simulink model "iface"  (R2018b)
settings: Solver=FixedStepDiscrete  StartTime=0.0  StopTime=10.0  RelTol=1e-3
settings Model: Creator=matlab  LastModifiedBy=matlab

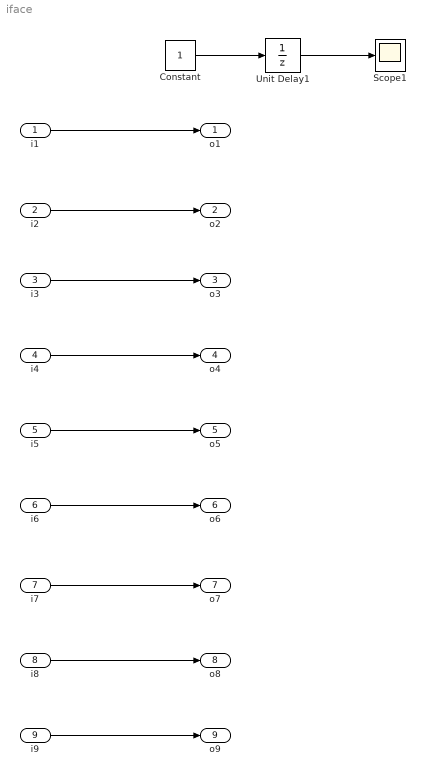
== system iface ==
  i1 : Inport  OutDataTypeStr=double  PortDimensions=[2 2]
  i2 : Inport  Port=2  OutDataTypeStr=single  PortDimensions=[2 2]
  i3 : Inport  Port=3  OutDataTypeStr=int8  PortDimensions=[2 2]
  i4 : Inport  Port=4  OutDataTypeStr=uint8  PortDimensions=[2 2]
  i5 : Inport  Port=5  OutDataTypeStr=int16  PortDimensions=[2 2]
  i6 : Inport  Port=6  OutDataTypeStr=uint16  PortDimensions=[2 2]
  i7 : Inport  Port=7  OutDataTypeStr=int32  PortDimensions=[2 2]
  i8 : Inport  Port=8  OutDataTypeStr=uint32  PortDimensions=[2 2]
  i9 : Inport  Port=9  OutDataTypeStr=boolean  PortDimensions=[2 2]
  Constant : Constant
  Scope1 : Scope
  Unit Delay1 : UnitDelay  SampleTime=-1
  o1 : Outport  OutDataTypeStr=double  PortDimensions=[2 2]
  o2 : Outport  Port=2  OutDataTypeStr=single  PortDimensions=[2 2]
  o3 : Outport  Port=3  OutDataTypeStr=int8  PortDimensions=[2 2]
  o4 : Outport  Port=4  OutDataTypeStr=uint8  PortDimensions=[2 2]
  o5 : Outport  Port=5  OutDataTypeStr=int16  PortDimensions=[2 2]
  o6 : Outport  Port=6  OutDataTypeStr=uint16  PortDimensions=[2 2]
  o7 : Outport  Port=7  OutDataTypeStr=int32  PortDimensions=[2 2]
  o8 : Outport  Port=8  OutDataTypeStr=uint32  PortDimensions=[2 2]
  o9 : Outport  Port=9  OutDataTypeStr=boolean  PortDimensions=[2 2]
  wires:
  i2/1 -> o2/1
  i3/1 -> o3/1
  i4/1 -> o4/1
  i5/1 -> o5/1
  i6/1 -> o6/1
  i7/1 -> o7/1
  i8/1 -> o8/1
  i9/1 -> o9/1
  i1/1 -> o1/1
  Unit Delay1/1 -> Scope1/1
  Constant/1 -> Unit Delay1/1
